simulink model "atomnedrustningv2"  (R2018b)
settings: Solver=VariableStepAuto  StartTime=0.0  StopTime=100.0  RelTol=1e-3
values from neighbouring files (symbols this model uses):
  nedrustningsavtale_rodnisser = 615    [parameeters.m]
  T1 = t    (= 1000)    [parameeters.m]
  T2 = t    (= 1000)    [parameeters.m]
  T3 = t    (= 1000)    [parameeters.m]
  T4 = t    (= 1000)    [parameeters.m]
settings Model: Creator=Magne Sirnes  LastModifiedBy=Magne Sirnes

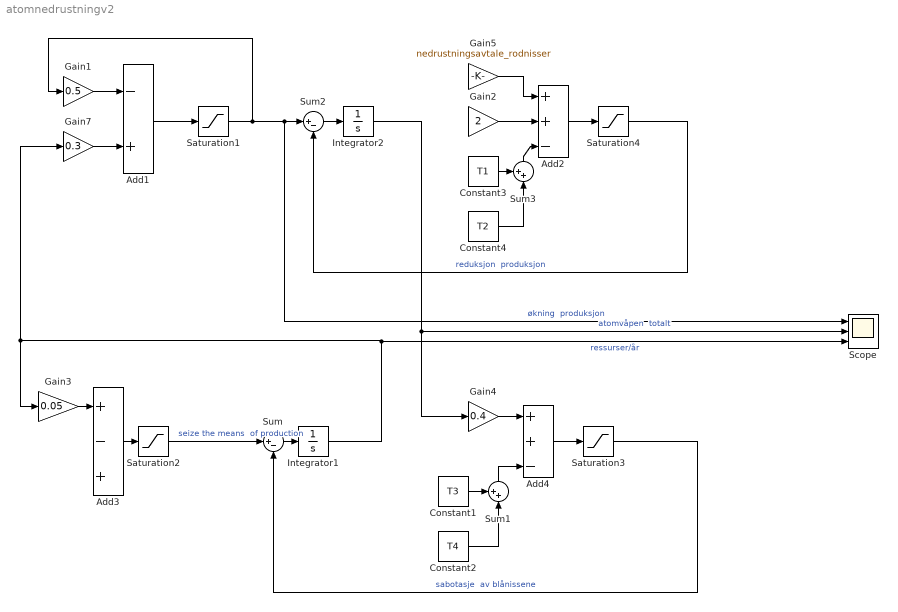
== system atomnedrustningv2 ==
  Add1 : Sum  Inputs=-+
  Add2 : Sum  Inputs=++-
  Add3 : Sum  Inputs=+-+
  Add4 : Sum  Inputs=++-
  Constant1 : Constant  Value=T3
  Constant2 : Constant  Value=T4
  Constant3 : Constant  Value=T1
  Constant4 : Constant  Value=T2
  Gain1 : Gain  Gain=0.5
  Gain2 : Gain  Gain=2
  Gain3 : Gain  Gain=0.05
  Gain4 : Gain  Gain=0.4
  Gain5 : Gain  Gain=nedrustningsavtale_rodnisser
  Gain7 : Gain  Gain=0.3
  Integrator1 : Integrator  InitialCondition=500  LimitOutput=on  LowerSaturationLimit=0
  Integrator2 : Integrator
  Saturation{1..4} (4 alike) : Saturate  UpperLimit=inf  LowerLimit=0
  Scope : Scope  NumInputPorts=3
  Sum : Sum  Inputs=|+-
  Sum1 : Sum  Inputs=++|
  Sum2 : Sum  Inputs=|+-
  Sum3 : Sum  Inputs=++|
  wires:
  Sum1/1 -> Add4/3
  Integrator1/1 -> Gain3/1, Gain7/1, Scope/3  "ressurser/år"
  Add4/1 -> Saturation3/1
  Constant1/1 -> Sum1/1
  Constant2/1 -> Sum1/2
  Saturation3/1 -> Sum/2  "sabotasje  av blånissene"
  Saturation2/1 -> Sum/1  "seize the means  of production"
  Add3/1 -> Saturation2/1
  Sum/1 -> Integrator1/1
  Integrator2/1 -> Scope/2, Gain4/1  "atomvåpen  totalt"
  Sum3/1 -> Add2/3
  Sum2/1 -> Integrator2/1
  Saturation4/1 -> Sum2/2  "reduksjon  produksjon"
  Gain5/1 -> Add2/1
  Gain7/1 -> Add1/2
  Add1/1 -> Saturation1/1
  Constant4/1 -> Sum3/2
  Saturation1/1 -> Gain1/1, Scope/1, Sum2/1  "økning  produksjon"
  Constant3/1 -> Sum3/1
  Add2/1 -> Saturation4/1
  Gain1/1 -> Add1/1
  Gain2/1 -> Add2/2
  Gain3/1 -> Add3/1
  Gain4/1 -> Add4/1
